simulink model "double_3D_pend_Euler_angles"  (R2024b)
settings: Solver=VariableStepAuto  StartTime=0.0  StopTime=4  FixedStep=0.01  MinStep=0.02  RelTol=1e-9  AbsTol=1e-9  EnableMultiTasking=on
InitFcn:
  | addpath MuscleForces\
  | addpath EquationsOfMotion\
  | initFunction
StopFcn:
  | % disp('Number simulation steps:')
  | % disp(length(out.tout))
  | 
  | line_colors = [0, 0, 1, 1; 1, 0, 0, 1;0, 1, 0, 1; 0.4660, 0.6740, 0.1880, 1];
  | line_colors_simulink = [0, 0, 1, 1; 1, 0, 0, 1;0, 1, 0, 1; 0.4660, 0.6740, 0.1880, 1];
  | time = out.tout;
  | time_interp = linspace(0,time(end),30);
  | time_GL = linspace(0,5,30);
  | GL_position = zeros(1,30);
  | yrot1 = out.yzy_1_eq.Data(1,:);
  | zrot1 = out.yzy_1_eq.Data(2,:);
  | xrot1 = out.yzy_1_eq.Data(3,:);
  | yrot_simulink1 = out.yzy_1.Data(1,:);
  | zrot_simulink1 = out.yzy_1.Data(2,:);
  | xrot_simulink1 = out.yzy_1.Data(3,:);
  | yrot_simulink_interp1 = interp1(time,yrot_simulink1,time_interp);
  | zrot_simulink_interp1 = interp1(time,zrot_simulink1,time_interp);
  | xrot_simulink_interp1 = interp1(time,xrot_simulink1,time_interp);
  | yrot2 = out.yzy_2_eq.Data(1,:);
  | zrot2 = out.yzy_2_eq.Data(2,:);
  | xrot2 = out.yzy_2_eq.Data(3,:);
  | yrot_simulink2 = out.yzy_2.Data(1,:);
  | zrot_simulink2 = out.yzy_2.Data(2,:);
  | xrot_simulink2 = out.yzy_2.Data(3,:);
  | yrot_simulink_interp2 = interp1(time,yrot_simulink2,time_interp);
  | zrot_simulink_interp2 = interp1(time,zrot_simulink2,time_interp);
  | xrot_simulink_interp2 = interp1(time,xrot_simulink2,time_interp);
  | 
  | figure
  | end_point = 1;
  | subplot(2,1,1)
  | plot(time(1:end-end_point),rad2deg(yrot1(1:end-end_point)),'LineWidth',1.5,'Color',line_colors_simulink(1,:)); hold on
  | plot(time(1:end-end_point),rad2deg(zrot1(1:end-end_point)),'LineWidth',1.5,'Color',line_colors_simulink(2,:)); hold on
  | plot(time(1:end-end_point),rad2deg(xrot1(1:end-end_point)),'LineWidth',1.5,'Color',line_colors_simulink(3,:)); hold on
  | plot(time_GL, GL_position,'LineWidth',1.5,'Color','k')
  | % plot(time_interp(1:end-end_point),rad2deg(yrot_simulink_interp1(1:end-end_point)),'Color',line_colors_simulink(1,:),'Marker','o','LineStyle', 'none','MarkerSize',8); hold on
  | % plot(time_interp(1:end-end_point),rad2deg(zrot_simulink_interp1(1:end-end_point)),'Color',line_colors_simulink(2,:),'Marker','o','LineStyle', 'none','MarkerSize',8); hold on
  | % plot(time_interp(1:end-end_point),rad2deg(xrot_simulink_interp1(1:end-end_point)),'Color',line_colors_simulink(3,:),'Marker','o','LineStyle', 'none','MarkerSize',8); hold on
  | 
  | hold off
  | xlim([0 4])
  | ylim([rad2deg(-2) rad2deg(3)])
  | % leg = legend({'R^{Y}','R^{Z}','R^{YY}',['Gimbal lock',newline, 'for YZY'],'R^{Y}_{Sim}','R^{Z}_{Sim}','R^{YY}_{Sim}'},'NumColumns',2,'FontSize',8,'Location','northeast');
  | leg = legend({'R_{Y}^{Upper}','R_{Z}^{Upper}','R_{YY}^{Upper}',['Gimbal lock',newline,'for YZY'],''},'NumColumns',1,'FontSize',8);
  | leg.IconColumnWidth = 10;
  | leg.Position(1) = [0.7];
  | leg.Position(2) = [0.68];
  | yticks([-90,0,90])
  | title('Euler angles-based model - Upper joint')
  | xlabel('Time [s]')
  | ylabel('Angle [deg]')
  | 
  | subplot(2,1,2)
  | plot(time(1:end-end_point),rad2deg(yrot2(1:end-end_point)),'LineWidth',1.5,'Color',line_colors_simulink(1,:)); hold on
  | plot(time(1:end-end_point),rad2deg(zrot2(1:end-end_point)),'LineWidth',1.5,'Color',line_colors_simulink(2,:)); hold on
  | plot(time(1:end-end_point),rad2deg(xrot2(1:end-end_point)),'LineWidth',1.5,'Color',line_colors_simulink(3,:)); hold on
  | plot(time_GL, ones(1,30)*(rad2deg(-pi/2)),time_GL, ones(1,30)*(rad2deg(pi/2)),'LineWidth',1.5,'Color','k')
  | % plot(time_interp(1:end-end_point),rad2deg(yrot_simulink_interp2(1:end-end_point)),'Color',line_colors_simulink(1,:),'Marker','o','LineStyle', 'none','MarkerSize',8); hold on
  | % plot(time_interp(1:end-end_point),rad2deg(zrot_simulink_interp2(1:end-end_point)),'Color',line_colors_simulink(2,:),'Marker','o','LineStyle', 'none','MarkerSize',8); hold on
  | % plot(time_interp(1:end-end_point),rad2deg(xrot_simulink_interp2(1:end-end_point)),'Color',line_colors_simulink(3,:),'Marker','o','LineStyle', 'none','MarkerSize',8); hold on
  | ... (+15 lines)
values from neighbouring files (symbols this model uses):
  activation = [0.1,0.5,0.1,0.1,0.1,0.1]    [data.m]    (also in initFunction.m = [0.1,1,0.1,1,0.1,0.1])
  eul1init = rotm2eul(rotm1init,"YZY")    [initFunction.m]
  fmax = [10,25,12,8,7,5]*1.2    [initFunction.m]
  lceopt = [2,2.3,1.2,1.5,2.5,2.1]    [initFunction.m]
  m = 1    [data.m]
  model =     [model_struct.mat]    (also in parameters.mat)
  out = sim("double_3D_pend_Quat.slx")    [plot_jacobian.m]
undefined symbols (not defined in the file or in its folder): initialConditions, X, Y, Z
libraries: sm_lib x37, nesl_utility x17
(part 2 of 2)

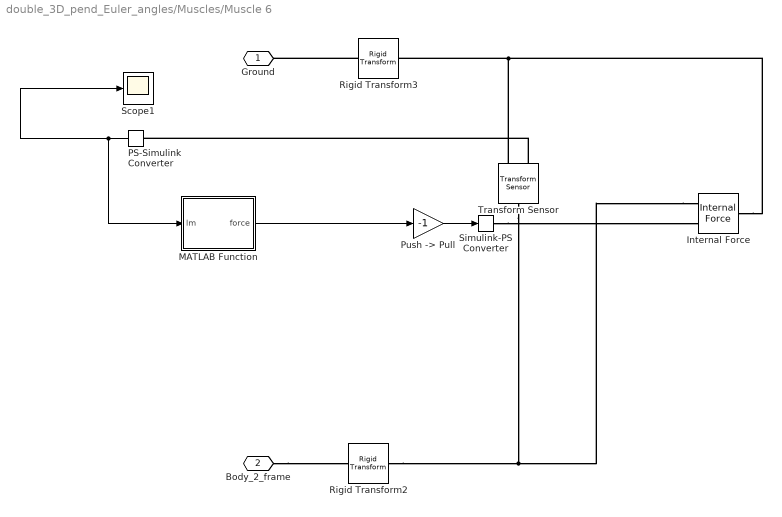
== system double_3D_pend_Euler_angles/Muscles/Muscle 6 ==
  Internal Force : sm_lib/Forces and Torques/Internal Force
  MATLAB Function : MATLAB Function  TreatAsAtomicUnit=on
  PS-Simulink Converter : nesl_utility/PS-Simulink Converter  PhysicalDomain=network_engine_domain  SubClassName=ps_output  LeftPortType=input  RightPortType=output  PseudoPeriodic=off  Frequencies=[]  VectorFormat=inherit  Unit=inherit  AffineConversion=off
  "Push -> Pull" : Gain  Gain=-1
  Rigid Transform2 : sm_lib/Frames and Transforms/Rigid Transform  RotationMethod=None  FollAlignAxisA=+X  BaseAlignAxisA=+Y  FollAlignAxisB=+Y  BaseAlignAxisB=+Z  RotationStandardAxis=+Z  RotationAngle=0.0  RotationAngleUnits=deg  RotationArbitraryAxis=[0 0 1]  RotationSequenceAxes=FollowerAxes  RotationSequence=XYX  RotationSequenceAngles=[0 0 0]  RotationSequenceAnglesUnits=deg  RotationMatrix=[1 0 0; 0 1 0; 0 0 1]  Quaternion=[1 0 0 0]  TranslationMethod=Cartesian  TranslationCartesianOffset=model.muscle6.insertion  TranslationCartesianOffsetUnits=m  TranslationStandardAxis=+Z  TranslationStandardOffset=0  TranslationStandardOffsetUnits=m  TranslationROffset=0  TranslationROffsetUnits=m  TranslationThetaOffset=0  TranslationThetaOffsetUnits=deg  TranslationZOffset=0  TranslationZOffsetUnits=m
  Rigid Transform3 : sm_lib/Frames and Transforms/Rigid Transform  RotationMethod=None  FollAlignAxisA=+X  BaseAlignAxisA=+Y  FollAlignAxisB=+Y  BaseAlignAxisB=+Z  RotationStandardAxis=+Z  RotationAngle=0.0  RotationAngleUnits=deg  RotationArbitraryAxis=[0 0 1]  RotationSequenceAxes=FollowerAxes  RotationSequence=XYX  RotationSequenceAngles=[0 0 0]  RotationSequenceAnglesUnits=deg  RotationMatrix=[1 0 0; 0 1 0; 0 0 1]  Quaternion=[1 0 0 0]  TranslationMethod=Cartesian  TranslationCartesianOffset=model.muscle6.origin  TranslationCartesianOffsetUnits=m  TranslationStandardAxis=+Z  TranslationStandardOffset=0  TranslationStandardOffsetUnits=m  TranslationROffset=0  TranslationROffsetUnits=m  TranslationThetaOffset=0  TranslationThetaOffsetUnits=deg  TranslationZOffset=0  TranslationZOffsetUnits=m
  Scope1 : Scope
  Simulink-PS Converter : nesl_utility/Simulink-PS Converter  PhysicalDomain=network_engine_domain  SubClassName=ps_input  LeftPortType=input  RightPortType=output  PseudoPeriodic=off  Frequencies=[]  NoiseDistribution=none  NoiseParameters=[]  Unit=1  AffineConversion=off  FilteringAndDerivatives=provide  SimscapeFilterOrder=1  InputFilterTimeConstant=0.001  UdotUserProvided=0
  Transform Sensor : sm_lib/Frames and Transforms/Transform Sensor  MeasurementFrame=World  RotationSequence=XYX  SenseAngle=off  SenseAxis=off  SenseQ=off  SenseR=off  SenseRotationSequence=off  SenseOmegaX=off  SenseOmegaY=off  SenseOmegaZ=off  SenseOmega=off  SenseQDot=off  SenseRDot=off  SenseRotationSequenceDot=off  SenseAlphaX=off  SenseAlphaY=off  SenseAlphaZ=off  SenseAlpha=off  SenseQDDot=off  SenseRDDot=off  SenseX=off  SenseY=off  SenseZ=off  SenseXYZ=off  SenseRad=off  SenseAzim=off  SenseDist=on  SenseInc=off  SenseXDot=off  SenseYDot=off  SenseZDot=off  SenseXYZDot=off  SenseRadDot=off  SenseAzimDot=off  SenseDistDot=off  SenseIncDot=off  SenseXDDot=off  SenseYDDot=off  SenseZDDot=off  SenseXYZDDot=off  SenseRadDDot=off  SenseAzimDDot=off  SenseDistDDot=off  SenseIncDDot=off
  Ground : PMIOPort  Side=Left
  Body_2_frame : PMIOPort  Port=2  Side=Left
  wires:
  "Push -> Pull"/1 -> Simulink-PS Converter/1
  MATLAB Function/1(force) -> "Push -> Pull"/1
  PS-Simulink Converter/1 -> MATLAB Function/1(lm), Scope1/1
  connections:
  Transform Sensor/RConn2 -- PS-Simulink Converter/LConn1
  Simulink-PS Converter/RConn1 -- Internal Force/LConn2
  Rigid Transform3/RConn1 -- Internal Force/RConn1 -- Transform Sensor/RConn1
  Internal Force/LConn1 -- Transform Sensor/LConn1 -- Rigid Transform2/RConn1
  Rigid Transform3/LConn1 -- Ground/RConn1
  Body_2_frame/RConn1 -- Rigid Transform2/LConn1

== matlab function double_3D_pend_Euler_angles/Muscles/Muscle 2/MATLAB Function ==
  data: force output; lm input; fmax parameter; lceopt parameter; activation parameter
function force = fcn(lm, fmax, lceopt, activation)

force = muscle_force(activation(2), lm, fmax(2), lceopt(2));

== matlab function double_3D_pend_Euler_angles/Muscles/Muscle 1/MATLAB Function ==
  data: force output; lm input; fmax parameter; lceopt parameter; activation parameter
function force = fcn(lm, fmax, lceopt, activation)

force = muscle_force(activation(1), lm, fmax(1), lceopt(1));

== matlab function double_3D_pend_Euler_angles/Muscles/Muscle 3/MATLAB Function ==
  data: force output; lm input; fmax parameter; lceopt parameter; activation parameter
function force = fcn(lm, fmax, lceopt, activation)

force = muscle_force(activation(3), lm, fmax(3), lceopt(3));

== matlab function double_3D_pend_Euler_angles/Muscles/Muscle 4/MATLAB Function ==
  data: force output; lm input; fmax parameter; lceopt parameter; activation parameter
function force = fcn(lm, fmax, lceopt, activation)

force = muscle_force(activation(4), lm, fmax(4), lceopt(4));

== matlab function double_3D_pend_Euler_angles/Muscles/Muscle 5/MATLAB Function ==
  data: force output; lm input; fmax parameter; lceopt parameter; activation parameter
function force = fcn(lm, fmax, lceopt, activation)

force = muscle_force(activation(5), lm, fmax(5), lceopt(5));

== matlab function double_3D_pend_Euler_angles/Muscles/Muscle 6/MATLAB Function ==
  data: force output; lm input; fmax parameter; lceopt parameter; activation parameter
function force = fcn(lm, fmax, lceopt, activation)

force = muscle_force(activation(6), lm, fmax(6), lceopt(6));

== matlab function double_3D_pend_Euler_angles/Dynamical_system ==
  data: u input; model parameter; y output; quat1T output; quat2T output; q1 output; q2 output; lceopt parameter; fmax parameter; act input
function [y,quat1T,quat2T,q1,q2] = fcn(u,model,lceopt, fmax, act)
t = 0;
y = zeros(12,1);
q1 = u(1:3);
q2 = u(4:6);

%recalculate to quaternions to compare with SimScape model
rotm1 = eul2rotm(q1','YZY');
quat1 = rotm2quat(rotm1);
quat1T = quat1';
rotm2 = eul2rotm(q2','YZX');
quat2 = rotm2quat(rotm2);
quat2T = quat2';
%generalized velocitites
u1 = u(7:9);
u2 = u(10:end);

FM = FM_eul(0,[q1;q2]',fmax,lceopt,act);
MM = mm_eul([q1;q2],[u1;u2],0,model);
FE = fo_eul([q1;q2],[u1;u2],0,model);
y = MM\(FE+[zeros(6,1);FM]);

end
